simulink model "Generic"  (R2018a)
settings: Solver=VariableStepAuto  StartTime=0.0  StopTime=.5  RelTol=1e-3  EnableMultiTasking=on
undefined symbols (not defined in the file): D1, Delta
libraries: powerlib x56
settings Model: Creator=AWAIS  LastModifiedBy=DELL
settings SolverCC: ZeroCrossAlgorithm=Adaptive
settings DataIOCC: LimitDataPoints=on  SaveFormat=Array
settings OptimizationCC: ExpressionDepthLimit=2147483647  LifeSpan=inf
settings DebuggingCC: UnderspecifiedInitializationDetection=Classic  MergeDetectMultiDrivingBlocksExec=none  MaxConsecutiveZCsMsg=none  SolverPrmCheckMsg=warning  StateNameClashWarn=warning  SFUnexpectedBacktrackingDiag=warning  SFNoUnconditionalDefaultTransitionDiag=warning  SFExecutionAtInitializationDiag=none
settings HardwareCC: ProdBitPerPointer=32  ProdBitPerSizeT=32  ProdBitPerPtrDiffT=32  ProdLargestAtomicFloat=None  ProdIntDivRoundTo=Undefined  ProdEndianess=Unspecified  ProdWordSize=32  ProdHWDeviceType=32-bit Generic
settings ModelReferenceCC: PropagateSignalLabelsOutOfModel=off
settings CodeAppCC: StateflowObjectComments=on
settings GRTTargetCC: TargetLangStandard=C89/C90 (ANSI)  GeneratePreprocessorConditionals=Disable all
settings ConfigComp: CovMetricSettings=dw  CovHtmlReporting=on  CovSaveCumulativeToWorkspaceVar=on  CovSaveSingleToWorkspaceVar=on  CovExternalEMLEnable=off
settings SimscapeCC: SimscapeNormalizeSystem=off

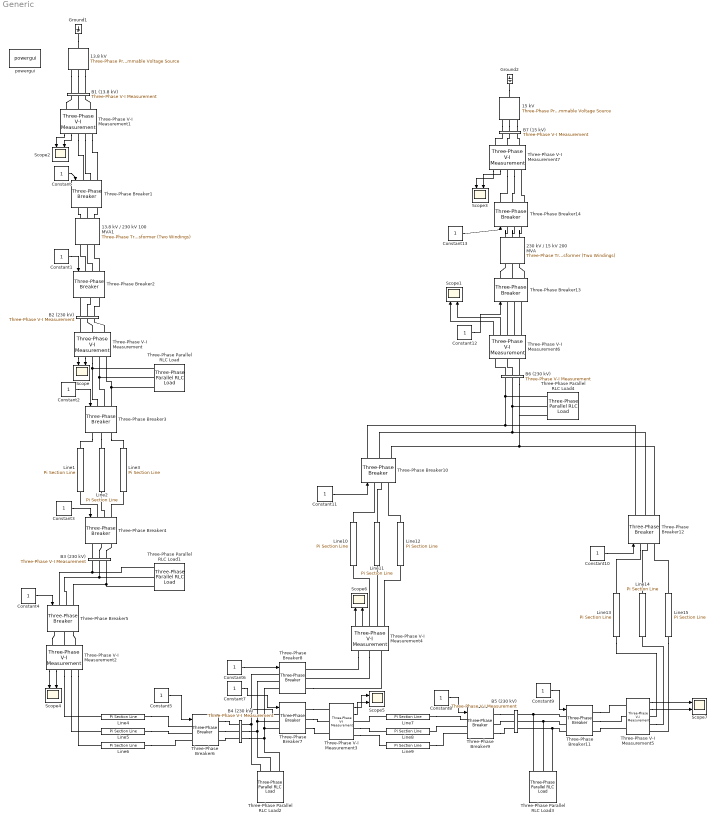
== system Generic ==
  13.8 kV : powerlib/Electrical Sources/Three-Phase Programmable Voltage Source  PositiveSequence=[13.8e3 0 60]  VariationEntity=Amplitude  VariationType=Table of time-amplitude pairs  VariationTypeAlt=Step  VariationStep=-0.2  VariationRate=10  VariationMagnitude=0.3  VariationFrequency=2  VariationTiming=[0.05 0.05+5/60]  VariationPhaseA=off  Amplitudes=[1 0.75 1.0]  TimeValues=[0 0.03 0.13]  HarmonicGeneration=off  HarmonicA=[1 -0.1 0 2]  HarmonicB=[2 0.15 35 2]*0  Timing="[0.1  2]"  BusType=PV  Pref=100e6  Qref=0  Qmin=-inf  Qmax=inf
  13.8 kV / 230 kV 100 MVA1 : powerlib/Elements/Three-Phase Transformer (Two Windings)  Winding1Connection=Delta (D1)  Winding2Connection=Yg  CoreType=Three single-phase transformers  SetSaturation=off  Hysteresis=off  DataFile='basic_model'  SetInitialFlux=off  Measurements=None  UNITS=pu  NominalPower=[100e6 60 ]  Winding1="[ 13.8e3  0.1/30   0.1 ]"  Winding2="[ 230e3  0.1/30  0.1]"  Rm=500  Lm=500  L0=0.5  Saturation="[ 0,0  ;  0.005,1.2  ;  1.0,1.4 ]"  InitialFluxes=[ 0.8 , -0.8 , 0.7 ]  MoreParameters=off  BreakLoop=off  DataType=off  TransfoNumber=0
  15 kV : powerlib/Electrical Sources/Three-Phase Programmable Voltage Source  PositiveSequence=[15e3 0 60]  VariationEntity=Amplitude  VariationType=Table of time-amplitude pairs  VariationTypeAlt=Step  VariationStep=-0.2  VariationRate=10  VariationMagnitude=0.3  VariationFrequency=2  VariationTiming=[0.05 0.05+5/60]  VariationPhaseA=off  Amplitudes=[1 0.75 1.0]  TimeValues=[0 0.03 0.13]  HarmonicGeneration=off  HarmonicA=[1 -0.1 0 2]  HarmonicB=[2 0.15 35 2]*0  Timing="[0.1  2]"  BusType=PQ  Pref=200e6  Qref=inf  Qmin=-inf  Qmax=inf
  230 kV / 15 kV 200 MVA : powerlib/Elements/Three-Phase Transformer (Two Windings)  Winding1Connection=Delta (D1)  Winding2Connection=Yg  CoreType=Three single-phase transformers  SetSaturation=off  Hysteresis=off  DataFile='basic_model'  SetInitialFlux=off  Measurements=None  UNITS=pu  NominalPower=[200e6 60 ]  Winding1="[ 15e3  0.1/30   0.1 ]"  Winding2="[ 230e3  0.1/30  0.1]"  Rm=500  Lm=500  L0=0.5  Saturation="[ 0,0  ;  0.005,1.2  ;  1.0,1.4 ]"  InitialFluxes=[ 0.8 , -0.8 , 0.7 ]  MoreParameters=off  BreakLoop=off  DataType=off  TransfoNumber=0
  B1 (13.8 kV) : powerlib/Measurements/Three-Phase V-I Measurement  VoltageMeasurement=no  SetLabelV=off  LabelV=Vabc_B120  Vpu=off  VpuLL=off  CurrentMeasurement=no  SetLabelI=on  LabelI=Iabc_B120  Ipu=off  Pbase=100e6  Vbase=120e3  OutputType=Complex  PhasorSimulation=off  PSBequivalent=0
  B2 (230 kV) : powerlib/Measurements/Three-Phase V-I Measurement  VoltageMeasurement=no  SetLabelV=off  LabelV=Vabc_B120  Vpu=off  VpuLL=off  CurrentMeasurement=no  SetLabelI=on  LabelI=Iabc_B120  Ipu=off  Pbase=100e6  Vbase=120e3  OutputType=Complex  PhasorSimulation=off  PSBequivalent=0
  B3 (230 kV) : powerlib/Measurements/Three-Phase V-I Measurement  VoltageMeasurement=no  SetLabelV=off  LabelV=Vabc_B120  Vpu=off  VpuLL=off  CurrentMeasurement=no  SetLabelI=on  LabelI=Iabc_B120  Ipu=off  Pbase=100e6  Vbase=120e3  OutputType=Complex  PhasorSimulation=off  PSBequivalent=0
  B4 (230 kV) : powerlib/Measurements/Three-Phase V-I Measurement  VoltageMeasurement=no  SetLabelV=off  LabelV=Vabc_B120  Vpu=off  VpuLL=off  CurrentMeasurement=no  SetLabelI=on  LabelI=Iabc_B120  Ipu=off  Pbase=100e6  Vbase=120e3  OutputType=Complex  PhasorSimulation=off  PSBequivalent=0
  B5 (230 kV) : powerlib/Measurements/Three-Phase V-I Measurement  VoltageMeasurement=no  SetLabelV=off  LabelV=Vabc_B120  Vpu=off  VpuLL=off  CurrentMeasurement=no  SetLabelI=on  LabelI=Iabc_B120  Ipu=off  Pbase=100e6  Vbase=120e3  OutputType=Complex  PhasorSimulation=off  PSBequivalent=0
  B6 (230 kV) : powerlib/Measurements/Three-Phase V-I Measurement  VoltageMeasurement=no  SetLabelV=off  LabelV=Vabc_B120  Vpu=off  VpuLL=off  CurrentMeasurement=no  SetLabelI=on  LabelI=Iabc_B120  Ipu=off  Pbase=100e6  Vbase=120e3  OutputType=Complex  PhasorSimulation=off  PSBequivalent=0
  B7 (15 kV) : powerlib/Measurements/Three-Phase V-I Measurement  VoltageMeasurement=no  SetLabelV=off  LabelV=Vabc_B120  Vpu=off  VpuLL=off  CurrentMeasurement=no  SetLabelI=on  LabelI=Iabc_B120  Ipu=off  Pbase=100e6  Vbase=120e3  OutputType=Complex  PhasorSimulation=off  PSBequivalent=0
  Constant{,1..13} (14 alike) : Constant
  Ground1 : powerlib/Elements/Ground  LConnTagsString=a
  Ground2 : powerlib/Elements/Ground  LConnTagsString=a
  Line{1..3,13..15} (6 alike) : powerlib/Elements/Pi Section Line  LConnTagsString=__new0  RConnTagsString=__new0  Frequency=50  Resistance=.08  Inductance=.0016  Capacitance=1e-6  Length=15  PiSections=2  Measurements=None
      settings: AttributesFormatString=\n  SourceProductName=Simscape Power Systems  SourceProductBaseCode=PS
  Line10 : powerlib/Elements/Pi Section Line  LConnTagsString=__new0  RConnTagsString=__new0  Frequency=50  Resistance=.08  Inductance=.0016  Capacitance=1e-6  Length=50  PiSections=2  Measurements=None
      settings: AttributesFormatString=\n  SourceProductName=Simscape Power Systems  SourceProductBaseCode=PS
  Line11 : powerlib/Elements/Pi Section Line  LConnTagsString=__new0  RConnTagsString=__new0  Frequency=50  Resistance=.08  Inductance=.0016  Capacitance=1e-6  Length=50  PiSections=2  Measurements=None
      settings: AttributesFormatString=\n  SourceProductName=Simscape Power Systems  SourceProductBaseCode=PS
  Line12 : powerlib/Elements/Pi Section Line  LConnTagsString=__new0  RConnTagsString=__new0  Frequency=50  Resistance=.08  Inductance=.0016  Capacitance=1e-6  Length=50  PiSections=2  Measurements=None
      settings: AttributesFormatString=\n  SourceProductName=Simscape Power Systems  SourceProductBaseCode=PS
  Line4 : powerlib/Elements/Pi Section Line  LConnTagsString=__new0  RConnTagsString=__new0  Frequency=50  Resistance=.08  Inductance=.0016  Capacitance=1e-6  Length=30  PiSections=2  Measurements=None
      settings: AttributesFormatString=\n  SourceProductName=Simscape Power Systems  SourceProductBaseCode=PS
  Line5 : powerlib/Elements/Pi Section Line  LConnTagsString=__new0  RConnTagsString=__new0  Frequency=50  Resistance=.08  Inductance=.0016  Capacitance=1e-6  Length=30  PiSections=2  Measurements=None
      settings: AttributesFormatString=\n  SourceProductName=Simscape Power Systems  SourceProductBaseCode=PS
  Line6 : powerlib/Elements/Pi Section Line  LConnTagsString=__new0  RConnTagsString=__new0  Frequency=50  Resistance=.08  Inductance=.0016  Capacitance=1e-6  Length=30  PiSections=2  Measurements=None
      settings: AttributesFormatString=\n  SourceProductName=Simscape Power Systems  SourceProductBaseCode=PS
  Line7 : powerlib/Elements/Pi Section Line  LConnTagsString=__new0  RConnTagsString=__new0  Frequency=50  Resistance=.08  Inductance=.0016  Capacitance=1e-6  Length=40  PiSections=2  Measurements=None
      settings: AttributesFormatString=\n  SourceProductName=Simscape Power Systems  SourceProductBaseCode=PS
  Line8 : powerlib/Elements/Pi Section Line  LConnTagsString=__new0  RConnTagsString=__new0  Frequency=50  Resistance=.08  Inductance=.0016  Capacitance=1e-6  Length=40  PiSections=2  Measurements=None
      settings: AttributesFormatString=\n  SourceProductName=Simscape Power Systems  SourceProductBaseCode=PS
  Line9 : powerlib/Elements/Pi Section Line  LConnTagsString=__new0  RConnTagsString=__new0  Frequency=50  Resistance=.08  Inductance=.0016  Capacitance=1e-6  Length=40  PiSections=2  Measurements=None
      settings: AttributesFormatString=\n  SourceProductName=Simscape Power Systems  SourceProductBaseCode=PS
  Scope{,1..7} (8 alike) : Scope  NumInputPorts=2
  Three-Phase Breaker{1..14} (14 alike) : powerlib/Elements/Three-Phase Breaker  InitialState=closed  SwitchA=on  SwitchB=on  SwitchC=on  SwitchTimes="[4/60  10/60]"  External=on  BreakerResistance=0.001  SnubberResistance=1e6  SnubberCapacitance=inf  Measurements=None
  Three-Phase Parallel RLC Load{,1..4} (5 alike) : powerlib/Elements/Three-Phase Parallel RLC Load  LConnTagsString=A|B|C  Configuration=Y (grounded)  NominalVoltage=230e3  Vabc=[1e3 1e3 1e3]  Vabcp=[1e3 1e3 1e3]  NominalFrequency=60  UnbalancedPower=off  ActivePower=50e3  InductivePower=30e3  CapacitivePower=0  Pabc=[10e3 9e3 11e3]  QLabc=[100 90 110]  QCabc=[100 90 110]  Pabcp=[10e3 9e3 11e3]  QLabcp=[100 90 110]  QCabcp=[100 90 110]  Measurements=None  LoadType=constant Z
  Three-Phase V-I Measurement{,1..7} (8 alike) : powerlib/Measurements/Three-Phase V-I Measurement  VoltageMeasurement=phase-to-phase  SetLabelV=off  LabelV=Vabc  Vpu=off  VpuLL=off  CurrentMeasurement=yes  SetLabelI=off  LabelI=Iabc  Ipu=off  Pbase=100e6  Vbase=500e3  OutputType=Complex  PhasorSimulation=off  PSBequivalent=0
  powergui : powerlib/powergui  Priority=1  SimulationMode=Continuous  SampleTime=50e-6  frequency=60  Iterations=50  frequencyindice=60  Pbase=100e6  ErrMax=1e-4  UnitsV=kV  UnitsW=MW  buscounter=0  FunctionMessages=off  echomessages=off  EnableUseOfTLC=off  CurrentSourceSwitches=off  DisableSnubberDevices=off  DisableRonSwitches=off  DisableVfSwitches=off  DisplayEquations=off  SolverType=Tustin/Backward Euler (TBE)  Interpol=off  ExternalGateDelay=off  methode=off  Ts=100  x0status=blocks  SPID=off  SwTol=0  HookPort=off  RestoreLinks=warning  ResistiveCurrentMeasurement=off  Frange=[0:2:500]  Ylog=off  Xlog=on  ShowGrid=off  save=off  variable=ZData  structure=0  ZoomFFT=off  StartTime=0.0  cycles=1  DisplayStyle=1  fundamental=60  FreqAxis=off  MaxFrequency=1000  frequencyindicesteady=1  RmsSteady=1  display=off
  wires:
  Three-Phase V-I Measurement/1 -> Scope/1
  Three-Phase V-I Measurement/2 -> Scope/2
  Three-Phase V-I Measurement1/2 -> Scope2/2
  Three-Phase V-I Measurement1/1 -> Scope2/1
  Three-Phase V-I Measurement2/1 -> Scope4/1
  Three-Phase V-I Measurement2/2 -> Scope4/2
  Three-Phase V-I Measurement3/1 -> Scope5/1
  Three-Phase V-I Measurement3/2 -> Scope5/2
  Three-Phase V-I Measurement4/1 -> Scope6/1
  Three-Phase V-I Measurement4/2 -> Scope6/2
  Three-Phase V-I Measurement5/1 -> Scope7/1
  Three-Phase V-I Measurement5/2 -> Scope7/2
  Three-Phase V-I Measurement6/2 -> Scope1/2
  Three-Phase V-I Measurement6/1 -> Scope1/1
  Three-Phase V-I Measurement7/2 -> Scope3/2
  Three-Phase V-I Measurement7/1 -> Scope3/1
  Constant/1 -> Three-Phase Breaker1/1
  Constant1/1 -> Three-Phase Breaker2/1
  Constant2/1 -> Three-Phase Breaker3/1
  Constant3/1 -> Three-Phase Breaker4/1
  Constant4/1 -> Three-Phase Breaker5/1
  Constant5/1 -> Three-Phase Breaker6/1
  Constant6/1 -> Three-Phase Breaker8/1
  Constant7/1 -> Three-Phase Breaker7/1
  Constant8/1 -> Three-Phase Breaker9/1
  Constant9/1 -> Three-Phase Breaker11/1
  Constant10/1 -> Three-Phase Breaker12/1
  Constant11/1 -> Three-Phase Breaker10/1
  Constant12/1 -> Three-Phase Breaker13/1
  Constant13/1 -> Three-Phase Breaker14/1
  connections:
  Ground1/LConn1 -- 13.8 kV/LConn1
  Three-Phase Breaker1/RConn3 -- 13.8 kV / 230 kV 100 MVA1/LConn3
  13.8 kV / 230 kV 100 MVA1/LConn2 -- Three-Phase Breaker1/RConn2
  Three-Phase Breaker1/RConn1 -- 13.8 kV / 230 kV 100 MVA1/LConn1
  Three-Phase Breaker2/LConn2 -- 13.8 kV / 230 kV 100 MVA1/RConn2
  B2 (230 kV)/LConn3 -- Three-Phase Breaker2/RConn3
  B2 (230 kV)/LConn1 -- Three-Phase Breaker2/RConn1
  B2 (230 kV)/LConn2 -- Three-Phase Breaker2/RConn2
  Three-Phase Breaker3/LConn2 -- Three-Phase V-I Measurement/RConn2 -- Three-Phase Parallel RLC Load/LConn2
  Three-Phase V-I Measurement/RConn1 -- Three-Phase Parallel RLC Load/LConn1 -- Three-Phase Breaker3/LConn1
  Three-Phase Breaker4/LConn3 -- Line3/RConn1
  Three-Phase Breaker4/LConn2 -- Line2/RConn1
  Three-Phase Breaker4/LConn1 -- Line1/RConn1
  B3 (230 kV)/LConn2 -- Three-Phase Breaker4/RConn2
  B3 (230 kV)/LConn1 -- Three-Phase Breaker4/RConn1
  B3 (230 kV)/LConn3 -- Three-Phase Breaker4/RConn3
  Three-Phase Breaker5/LConn3 -- B3 (230 kV)/RConn3 -- Three-Phase Parallel RLC Load1/LConn3
  Three-Phase Breaker5/LConn2 -- Three-Phase Parallel RLC Load1/LConn2 -- B3 (230 kV)/RConn2
  Three-Phase Breaker5/LConn1 -- Three-Phase Parallel RLC Load1/LConn1 -- B3 (230 kV)/RConn1
  Line4/RConn1 -- Three-Phase Breaker6/LConn1
  Line5/RConn1 -- Three-Phase Breaker6/LConn2
  Line6/RConn1 -- Three-Phase Breaker6/LConn3
  Three-Phase Breaker6/RConn2 -- B4 (230 kV)/RConn2
  Three-Phase Breaker6/RConn3 -- B4 (230 kV)/RConn3
  Three-Phase Breaker6/RConn1 -- B4 (230 kV)/RConn1
  B4 (230 kV)/LConn3 -- Three-Phase Parallel RLC Load2/LConn3 -- Three-Phase Breaker7/LConn3 -- Three-Phase Breaker8/LConn3
  B4 (230 kV)/LConn2 -- Three-Phase Parallel RLC Load2/LConn2 -- Three-Phase Breaker7/LConn2 -- Three-Phase Breaker8/LConn2
  B4 (230 kV)/LConn1 -- Three-Phase Parallel RLC Load2/LConn1 -- Three-Phase Breaker8/LConn1 -- Three-Phase Breaker7/LConn1
  Line9/RConn1 -- Three-Phase Breaker9/LConn3
  Line8/RConn1 -- Three-Phase Breaker9/LConn2
  Line7/RConn1 -- Three-Phase Breaker9/LConn1
  Three-Phase Breaker10/LConn2 -- Line11/RConn1
  Line10/RConn1 -- Three-Phase Breaker10/LConn1
  Line12/RConn1 -- Three-Phase Breaker10/LConn3
  Three-Phase Breaker9/RConn2 -- B5 (230 kV)/RConn2
  Three-Phase Breaker9/RConn3 -- B5 (230 kV)/RConn3
  Three-Phase Breaker9/RConn1 -- B5 (230 kV)/RConn1
  Three-Phase Breaker11/LConn1 -- B5 (230 kV)/LConn1 -- Three-Phase Parallel RLC Load3/LConn1
  Three-Phase Breaker11/LConn2 -- Three-Phase Parallel RLC Load3/LConn2 -- B5 (230 kV)/LConn2
  Three-Phase Breaker11/LConn3 -- Three-Phase Parallel RLC Load3/LConn3 -- B5 (230 kV)/LConn3
  Three-Phase Breaker12/LConn2 -- Line14/RConn1
  Line15/RConn1 -- Three-Phase Breaker12/LConn3
  Three-Phase Breaker12/LConn1 -- Line13/RConn1
  Three-Phase Breaker10/RConn3 -- B6 (230 kV)/LConn3 -- Three-Phase Parallel RLC Load4/LConn3 -- Three-Phase Breaker12/RConn3
  Three-Phase Breaker10/RConn2 -- Three-Phase Breaker12/RConn2 -- Three-Phase Parallel RLC Load4/LConn2 -- B6 (230 kV)/LConn2
  Three-Phase Breaker10/RConn1 -- Three-Phase Breaker12/RConn1 -- Three-Phase Parallel RLC Load4/LConn1 -- B6 (230 kV)/LConn1
  Three-Phase Breaker13/RConn2 -- 230 kV / 15 kV 200 MVA/RConn2
  Three-Phase Breaker13/RConn3 -- 230 kV / 15 kV 200 MVA/RConn3
  Three-Phase Breaker13/RConn1 -- 230 kV / 15 kV 200 MVA/RConn1
  230 kV / 15 kV 200 MVA/LConn3 -- Three-Phase Breaker14/LConn3
  230 kV / 15 kV 200 MVA/LConn2 -- Three-Phase Breaker14/LConn2
  230 kV / 15 kV 200 MVA/LConn1 -- Three-Phase Breaker14/LConn1
  15 kV/RConn3 -- B7 (15 kV)/RConn3
  15 kV/RConn2 -- B7 (15 kV)/RConn2
  Ground2/LConn1 -- 15 kV/LConn1
  15 kV/RConn1 -- B7 (15 kV)/RConn1
  13.8 kV/RConn3 -- B1 (13.8 kV)/LConn3
  13.8 kV/RConn2 -- B1 (13.8 kV)/LConn2
  13.8 kV/RConn1 -- B1 (13.8 kV)/LConn1
  Three-Phase Breaker2/LConn1 -- 13.8 kV / 230 kV 100 MVA1/RConn1
  Three-Phase Breaker2/LConn3 -- 13.8 kV / 230 kV 100 MVA1/RConn3
  Three-Phase V-I Measurement/LConn3 -- B2 (230 kV)/RConn3
  Three-Phase V-I Measurement/LConn2 -- B2 (230 kV)/RConn2
  Three-Phase V-I Measurement/LConn1 -- B2 (230 kV)/RConn1
  Three-Phase V-I Measurement1/LConn3 -- B1 (13.8 kV)/RConn3
  Three-Phase V-I Measurement1/LConn2 -- B1 (13.8 kV)/RConn2
  Three-Phase V-I Measurement1/LConn1 -- B1 (13.8 kV)/RConn1
  Three-Phase V-I Measurement1/RConn3 -- Three-Phase Breaker1/LConn3
  Three-Phase V-I Measurement1/RConn2 -- Three-Phase Breaker1/LConn2
  Three-Phase V-I Measurement1/RConn1 -- Three-Phase Breaker1/LConn1
  Three-Phase V-I Measurement2/LConn2 -- Three-Phase Breaker5/RConn2
  Three-Phase V-I Measurement2/LConn3 -- Three-Phase Breaker5/RConn3
  Three-Phase V-I Measurement2/LConn1 -- Three-Phase Breaker5/RConn1
  Three-Phase V-I Measurement2/RConn1 -- Line4/LConn1
  Three-Phase V-I Measurement2/RConn2 -- Line5/LConn1
  Three-Phase V-I Measurement2/RConn3 -- Line6/LConn1
  Three-Phase Breaker7/RConn2 -- Three-Phase V-I Measurement3/LConn2
  Three-Phase Breaker7/RConn3 -- Three-Phase V-I Measurement3/LConn3
  Three-Phase Breaker7/RConn1 -- Three-Phase V-I Measurement3/LConn1
  Line7/LConn1 -- Three-Phase V-I Measurement3/RConn1
  Three-Phase V-I Measurement3/RConn2 -- Line8/LConn1
  Three-Phase V-I Measurement3/RConn3 -- Line9/LConn1
  Three-Phase V-I Measurement4/LConn1 -- Three-Phase Breaker8/RConn1
  Three-Phase V-I Measurement4/LConn2 -- Three-Phase Breaker8/RConn2
  Three-Phase Breaker8/RConn3 -- Three-Phase V-I Measurement4/LConn3
  Three-Phase V-I Measurement4/RConn3 -- Line12/LConn1
  Three-Phase V-I Measurement4/RConn2 -- Line11/LConn1
  Three-Phase V-I Measurement4/RConn1 -- Line10/LConn1
  Three-Phase Breaker11/RConn1 -- Three-Phase V-I Measurement5/LConn1
  Three-Phase Breaker11/RConn2 -- Three-Phase V-I Measurement5/LConn2
  Three-Phase Breaker11/RConn3 -- Three-Phase V-I Measurement5/LConn3
  Line13/LConn1 -- Three-Phase V-I Measurement5/RConn1
  Three-Phase V-I Measurement5/RConn2 -- Line14/LConn1
  Line15/LConn1 -- Three-Phase V-I Measurement5/RConn3
  B6 (230 kV)/RConn1 -- Three-Phase V-I Measurement6/LConn1
  B6 (230 kV)/RConn2 -- Three-Phase V-I Measurement6/LConn2
  B6 (230 kV)/RConn3 -- Three-Phase V-I Measurement6/LConn3
  Three-Phase V-I Measurement6/RConn3 -- Three-Phase Breaker13/LConn3
  Three-Phase V-I Measurement6/RConn2 -- Three-Phase Breaker13/LConn2
  Three-Phase V-I Measurement6/RConn1 -- Three-Phase Breaker13/LConn1
  Three-Phase Breaker14/RConn3 -- Three-Phase V-I Measurement7/RConn3
  Three-Phase V-I Measurement7/RConn2 -- Three-Phase Breaker14/RConn2
  Three-Phase V-I Measurement7/RConn1 -- Three-Phase Breaker14/RConn1
  Three-Phase V-I Measurement7/LConn3 -- B7 (15 kV)/LConn3
  Three-Phase V-I Measurement7/LConn2 -- B7 (15 kV)/LConn2
  Three-Phase V-I Measurement7/LConn1 -- B7 (15 kV)/LConn1
  Three-Phase Breaker3/RConn3 -- Line3/LConn1
  Three-Phase Breaker3/RConn2 -- Line2/LConn1
  Three-Phase Breaker3/RConn1 -- Line1/LConn1
  Three-Phase Breaker3/LConn3 -- Three-Phase Parallel RLC Load/LConn3 -- Three-Phase V-I Measurement/RConn3
